simulink model "Reaching12"  (R2022b)
settings: Solver=FixedStepDiscrete  StartTime=0.0  StopTime=200  FixedStep=0.001  RelTol=1e-3
libraries: PhanTorque_3Dof_Library_64Bits x1, vrlib x1
settings Model: Creator=carlos.aldana  LastModifiedBy=Ammar Arsi
settings SolverCC: AlgebraicLoopSolver=TrustRegion
settings DataIOCC: LimitDataPoints=on  SaveFormat=Array  ReturnWorkspaceOutputs=off
settings OptimizationCC: BlockReduction=off  BooleanDataType=off  LifeSpan=inf
settings DebuggingCC: SaveWithParameterizedLinksMsg=none  UnderspecifiedInitializationDetection=Classic  MergeDetectMultiDrivingBlocksExec=none  SignalResolutionControl=TryResolveAllWithWarning  UnconnectedInputMsg=warning  UnconnectedOutputMsg=warning  UnconnectedLineMsg=warning  AllowSymbolicDim=off  SFUnexpectedBacktrackingDiag=warning  SFNoUnconditionalDefaultTransitionDiag=warning  SFExecutionAtInitializationDiag=none  SFMachineParentedDataDiag=warning  ArithmeticOperatorsInVariantConditions=warning
settings HardwareCC: ProdBitPerPointer=32  ProdBitPerSizeT=32  ProdBitPerPtrDiffT=32  ProdLargestAtomicFloat=None  ProdIntDivRoundTo=Undefined  ProdEndianess=Unspecified  ProdWordSize=32  ProdHWDeviceType=32-bit Generic  TargetUnknown=on
settings ModelReferenceCC: EnableRefExpFcnMdlSchedulingChecks=on  PropagateSignalLabelsOutOfModel=off
settings SFSimCC: SimUseLocalCustomCode=off  CustomCodeUndefinedFunction=UseInterfaceOnly
settings RTWCC: RTWUseLocalCustomCode=off  DLArmComputeVersion=19.05
settings CodeAppCC: StateflowObjectComments=on
settings GRTTargetCC: TargetLangStandard=C89/C90 (ANSI)
settings ConfigComp: CovMetricSettings=dw  CovSaveCumulativeToWorkspaceVar=on  CovSaveSingleToWorkspaceVar=on  CovExternalEMLEnable=off  CovSFcnEnable=off

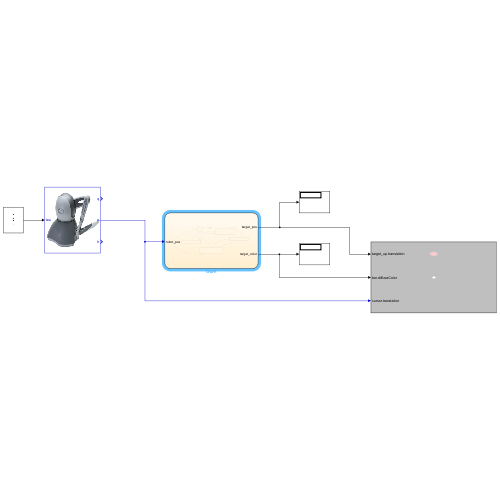
[thumbnail: Simulink's stored preview of the top-level diagram]
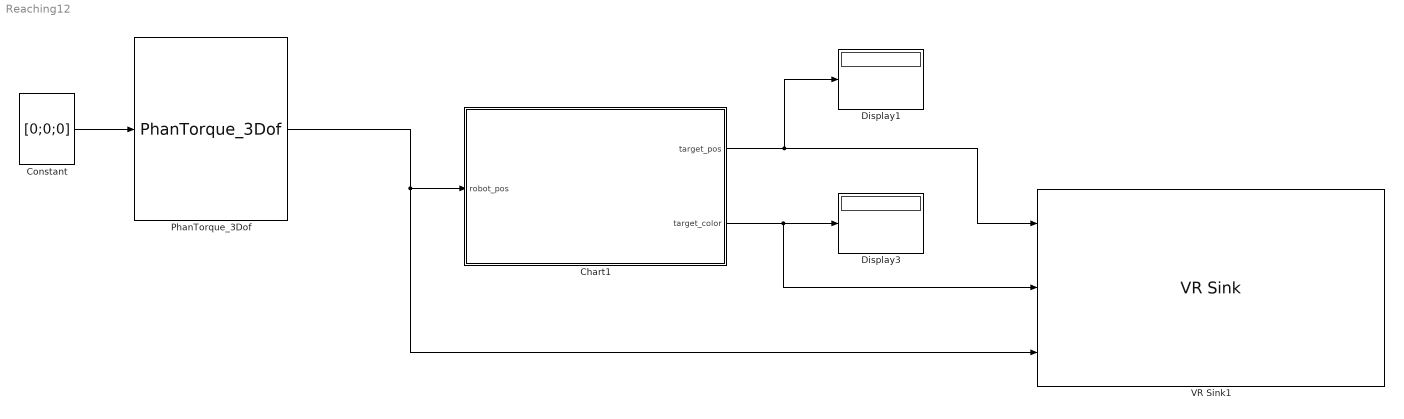
== system Reaching12 ==
  Chart1 : Stateflow chart  TreatAsAtomicUnit=on
  Constant : Constant  Value=[0;0;0]  VectorParams1D=off
  Display1 : Display
  Display3 : Display
  PhanTorque_3Dof : PhanTorque_3Dof_Library_64Bits/PhanTorque_3Dof  Haptic_Name='Default Device'
  VR Sink1 : vrlib/VR Sink  InstantiateOnLoad=on  SampleTime=0.1  ViewEnable=on  RemoteChange=off  RemoteView=off  FieldsWritten=target_up.translation.3.1.1.double#ber.diffuseColor.3.1.1.double#cursor.translation.3.1.1.double  WorldFileName=8test.wrl  AutoView=off  VideoDimensions=[]  AllowVariableSize=off
  wires:
  Chart1/1(target_pos) -> Display1/1, VR Sink1/1
  Chart1/2(target_color) -> VR Sink1/2, Display3/1
  Constant/1 -> PhanTorque_3Dof/1
  PhanTorque_3Dof/2 -> Chart1/1(robot_pos), VR Sink1/3

== stateflow chart Reaching12/Chart1 ==
  state Start
    entry:
    radius = 0.1;
    threshold = 0.01;
    target_color = [0 0 1];
    i = 1;
    target_pos = [0; 0; 0];
  state Finish
  note: angle could aslo be angle =2*pi/8
  state Target
    entry:
    target_color = [1 1 1];
    target_pos = [radius*cos(angle); radius*sin(angle); 0];
    distance_diff = (robot_pos(1,1)-target_pos(1,1))^2 +(robot_pos(2,1)-target_pos(2,1))^2;
    distance = sqrt(distance_diff);
    during:
    distance_diff = (robot_pos(1,1)-target_pos(1,1))^2 +(robot_pos(2,1)-target_pos(2,1))^2;
    distance = sqrt(distance_diff);
  state Colour_change_two
    entry:
    target_color = [1 0 0];
    during:
    distance_diff = (robot_pos(1,1)-target_pos(1,1))^2 +(robot_pos(2,1)-target_pos(2,1))^2;
    distance = sqrt(distance_diff);
  state Colour_1
    target_color = [1 0 1];
    during:
    distance_diff = (robot_pos(1,1)-target_pos(1,1))^2 +(robot_pos(2,1)-target_pos(2,1))^2;
    distance = sqrt(distance_diff);
  state Hometarget
    target_pos = [0; 0; 0];
    target_color = [0 0 1];
    distance_diff =  (robot_pos(1,1)-target_pos(1,1))^2 +(robot_pos(2,1)-target_pos(2,1))^2;
    distance = sqrt(distance_diff);
    during:
    distance_diff =  (robot_pos(1,1)-target_pos(1,1))^2 +(robot_pos(2,1)-target_pos(2,1))^2;
    distance = sqrt(distance_diff);
  Start -> Finish [order 2] : [i >= 10]
  Colour_change_two -> Target [order 1] : [after(2,sec) && distance<threshold]{angle = 2*pi*rand;}
  Start -> Hometarget [order 1] : [i <10]
  (default) -> Start
  Colour_1 -> Target [order 2] : [distance>threshold]
  Target -> Colour_1 : [distance<threshold]
  Hometarget -> Colour_change_two : [distance<threshold]
  Colour_1 -> Hometarget [order 1] : [after(1,sec) && distance<threshold]{i = i + 1;}
  Colour_change_two -> Hometarget [order 2] : [distance>threshold]
  data: target_pos output; target_color output; robot_pos input; angle local; distance local; i local; distance_diff local; threshold local double; radius local
